simulink model "sampleModel182"  (R2021b)
settings: Solver=VariableStepAuto  StartTime=0.0  StopTime=10.0  RelTol=1e-3
undefined symbols (not defined in the file or in its folder): DiscIntNeverNeededParam
libraries: simulink x26, slpidlib x2, simulink_need_slupdate x2
settings Model: Creator=user  LastModifiedBy=user

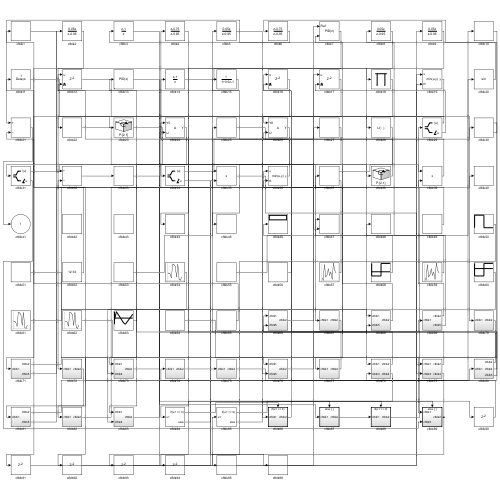
[thumbnail: Simulink's stored preview of the top-level diagram]
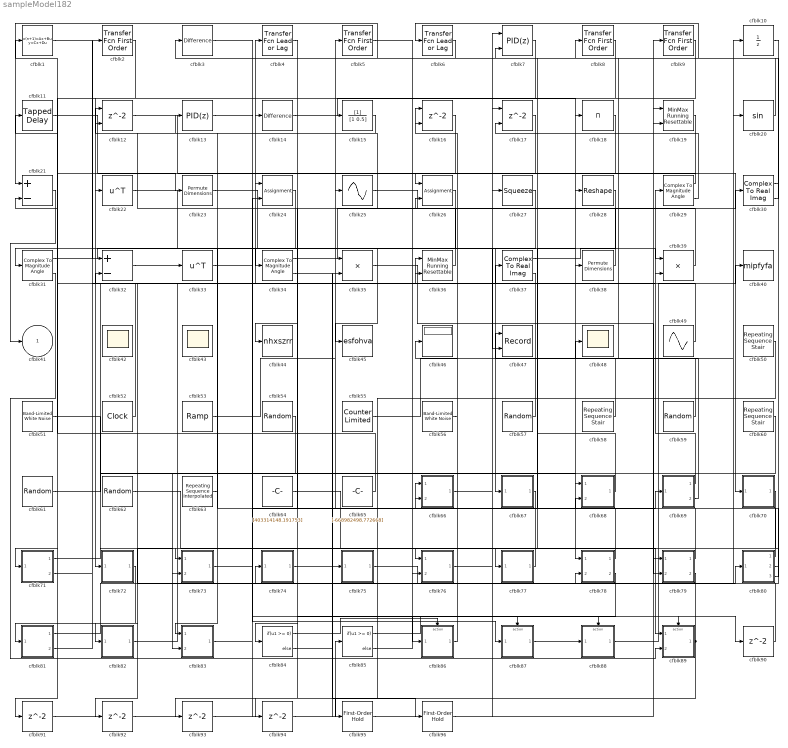
== system sampleModel182 ==
  cfblk1 : DiscreteStateSpace
  cfblk10 : UnitDelay  HasFrameUpgradeWarning=on
  cfblk11 : simulink/Discrete/Tapped Delay  vinit=0.0  samptime=-1  NumDelays=1  DelayOrder=Oldest  includeCurrent=off
  cfblk12 : Delay  ShowEnablePort=on  SampleTime=1
      settings: InputPortMap=u0,e6
  cfblk13 : slpidlib/PID Controller  Controller=PID  Form=Parallel  TimeDomain=Discrete-time  UseExternalTs=off  SampleTime=1  IntegratorMethod=Forward Euler  FilterMethod=Forward Euler  ControllerParametersSource=internal  P=1  I=1  D=0  UseFilter=on  N=100  TunerSelectOption=Transfer Function Based (PID Tuner App)  InitialConditionSource=internal  InitialConditionForIntegrator=0  InitialConditionForFilter=0  DifferentiatorICPrevScaledInput=0  ExternalReset=none  TrackingMode=off  Kt=1  LimitOutput=off  SatLimitsSource=internal  UpperSaturationLimit=inf  LowerSaturationLimit=-inf  LinearizeAsGain=off  AntiWindupMode=none  Kb=1  POutMin=[]  POutMax=[]  IOutMin=[]  IOutMax=[]  DOutMin=[]  DOutMax=[]  NOutMin=[]  NOutMax=[]  SumOutMin=[]  SumOutMax=[]  SaturationOutMin=[]  SaturationOutMax=[]  PParamMin=[]  PParamMax=[]  IParamMin=[]  IParamMax=[]  DParamMin=[]  DParamMax=[]  NParamMin=[]  NParamMax=[]  KbParamMin=[]  KbParamMax=[]  KtParamMin=[]  KtParamMax=[]  KbOutMin=[]  KbOutMax=[]  KtOutMin=[]  KtOutMax=[]  IntegratorOutMin=[]  IntegratorOutMax=[]  FilterOutMin=[]  FilterOutMax=[]  SumI1OutMin=[]  SumI1OutMax=[]  SumI2OutMin=[]  SumI2OutMax=[]  SumI3OutMin=[]  SumI3OutMax=[]  SumI4OutMin=[]  SumI4OutMax=[]  SumDOutMin=[]  SumDOutMax=[]  DifferentiatorOutMin=[]  DifferentiatorOutMax=[]  FilterDiffOutCoefMin=[]  FilterDiffOutCoefMax=[]  ReciprocalOutMin=[]  ReciprocalOutMax=[]  SumDenOutMin=[]  SumDenOutMax=[]  SumNumOutMin=[]  SumNumOutMax=[]  DivideOutMin=[]  DivideOutMax=[]  UdiffTsProdOutMin=[]  UdiffTsProdOutMax=[]  NTsProdOutMin=[]  NTsProdOutMax=[]  UintegralTsProdOutMin=[]  UintegralTsProdOutMax=[]  UngainTsProdOutMin=[]  UngainTsProdOutMax=[]  IntegratorContinuousStateAttributes=''  IntegratorStateMustResolveToSignalObject=off  IntegratorRTWStateStorageClass=Auto  FilterContinuousStateAttributes=''  FilterStateMustResolveToSignalObject=off  FilterRTWStateStorageClass=Auto  ParallelPVariant=InternalParameters  IdealPVariant=Disabled  IVariant=InternalParameters  DVariant=InternalParameters  IntegratorVariant=Discrete  SatVariant=Disabled  AWVariant=Passthrough  PCopyVariant=Disabled  TRVariant=Disabled  FdbkBlocksVariant=Forward  IdealPFdbkVariant=Disabled  SatFdbkVariant=Disabled  DerivativeFilterVariant=ForwardEulerFilter  NVariant=InternalParameters  NCopyVariant=Disabled  FilterICVariant=InternalICsFilter  IntegratorICVariant=InternalICs  ExternalResetVariant=Disabled  TRSumVariant=Passthrough  SumFdbkVariant=Disabled  SumVariant=Sum_PID  TsampFilterVariant=InternalTs  TsampNgainVariant=Passthrough  TsampIntegralVariant=Passthrough  ExternalSaturationOutDataTypeStr=Inherit: Same as second input
  cfblk14 : simulink/Discrete/Difference  ICPrevInput=0.0  OutMin=[]  OutMax=[]  OutDataTypeStr=Inherit: Inherit via back propagation  OutDataType=fixdt(1, 16)  OutScaling=2^-10  DoSatur=off
  cfblk15 : DiscreteFilter  SampleTime=1
  cfblk16 : Delay  ShowEnablePort=on  SampleTime=1
      settings: InputPortMap=u0,e6
  cfblk17 : Delay  ShowEnablePort=on  SampleTime=1
      settings: InputPortMap=u0,e6
  cfblk18 : Product  Inputs=*
  cfblk19 : simulink/Math Operations/MinMax Running Resettable  Function=min  vinit=0.0
  cfblk{2,5,8..9} (4 alike) : simulink/Discrete/Transfer Fcn First Order  PoleZ=0.95  ICPrevOutput=0.0  DoSatur=off
  cfblk20 : Trigonometry
  cfblk21 : Sum  Inputs=+-
  cfblk22 : Math  Operator=transpose  SaturateOnIntegerOverflow=on
  cfblk23 : PermuteDimensions
  cfblk24 : Assignment  DiagnosticForDimensions=Warning  IndexOptions=Index vector (dialog)  Indices=1  OutputSizes=1
  cfblk25 : Sin  TimeSource=Use external signal  SampleTime=0
  cfblk26 : Assignment  DiagnosticForDimensions=Warning  IndexOptions=Index vector (dialog)  Indices=1  OutputSizes=1
  cfblk27 : Squeeze
  cfblk28 : Reshape
  cfblk29 : ComplexToMagnitudeAngle
  cfblk3 : simulink/Discrete/Difference  ICPrevInput=0.0  OutMin=[]  OutMax=[]  OutDataTypeStr=Inherit: Inherit via back propagation  OutDataType=fixdt(1, 16)  OutScaling=2^-10  DoSatur=off
  cfblk30 : ComplexToRealImag
  cfblk31 : ComplexToMagnitudeAngle
  cfblk32 : Sum  Inputs=+-
  cfblk33 : Math  Operator=transpose  SaturateOnIntegerOverflow=on
  cfblk34 : ComplexToMagnitudeAngle
  cfblk35 : Product  Inputs=**
  cfblk36 : simulink/Math Operations/MinMax Running Resettable  Function=min  vinit=0.0
  cfblk37 : ComplexToRealImag
  cfblk38 : PermuteDimensions
  cfblk39 : Product
  cfblk4 : simulink/Discrete/Transfer Fcn Lead or Lag  PoleZ=0.95  ZeroZ=0.75  ICPrevOutput=0.0  ICPrevInput=0.0  DoSatur=off
      settings: SourceProductBaseCode=SL
  cfblk40 : ToWorkspace  VariableName=mipfyfa  SaveFormat=Timeseries  SampleTime=-1
  cfblk42 : Scope
      settings: Floating=on
  cfblk43 : Scope
      settings: Floating=on
  cfblk44 : ToWorkspace  VariableName=nhxszrr  SaveFormat=Timeseries  SampleTime=-1
  cfblk45 : ToWorkspace  VariableName=esfohva  SaveFormat=Timeseries  SampleTime=-1
  cfblk46 : Display
  cfblk47 : Record  FileSettingsInternal="{\"entries\":[{\"content\":{\"excelSettings\":{\"content\":{},\"type\":\"Streamout.ExcelSettings\"}},\"type\":\"Streamout.FileSettingStorage\",\"uuid\":\"d13ae737-717a-44e4-beef-aca473ab83c8\"}],\"packageUris\":[\"http://schema.mathworks.com/mf0/streamout_blocks/R2020a\"],\"version\":\"1.0\"}"  Layout=[1 1]  SignalsInternal="{\"entries\":[{\"content\":{\"signals\":[{\"content\":{\"blockPath\":[\"sampleModel182/cfblk47\"],\"channel\":[],\"dimensions\":[1],\"domain\":\"sampleModel182/cfblk47\",\"lineColor\":\"#a2142f\",\"plots\":[1],\"port\":1,\"sid\":[\"\"],\"signalID\":6832,\"signalName\":\"cfblk58\"},\"type\":\"RecordBlkView.Signal\",\"uuid\":\"52de0a0e-42b8-4ab6-a928-dbb1bce8dd43\"},{\"content\":{\"blockPath\":[\"sampleModel182/cfblk47\"],\"channel\":[],\"dimensions\":[1,1],\"domain\":\"sampleModel182/cfblk47\",\"lineColor\":\"#139fff\",\"plots\":[1],\"port\":2,\"sid\":[\"\"],\"signalID\":6836,\"signalName\":\"cfblk23\"},\"type\":\"RecordBlkView.Signal\",\"uuid\":\"73905647-726a-4450-a034-1e1480183f6b\"}]},\"type\":\"RecordBlkView.InputSignals\",\"uuid\":\"f9e11d63-c08c-4043-8374-cec281b00203\"}],\"packageUris\":[\"http://schema.mathworks.com/mf0/streamout_blocks/R2020a\"],\"version\":\"1.0\"}"  VisualizationBindings="{\"xyplotplugin\":{\"info\":[{\"series\":[{\"bindingParametersList\":[{\"parameter\":\"X-Axis\",\"signalID\":6832,\"signalName\":\"cfblk58\"},{\"parameter\":\"Y-Axis\",\"signalID\":6836,\"signalName\":\"cfblk23\"}],\"seriesID\":60133}],\"subplotID\":1}]}}"  CompatibilityTag=XY
  cfblk48 : Scope
  cfblk49 : Sin  Amplitude=[-141875672.299204]  Bias=[779859813.343924]  SampleTime=0
  cfblk50 : simulink/Sources/Repeating Sequence Stair  OutValues=[-60441637.723596, -585056576.833812]  tsamp=-1  OutMin=[]  OutMax=[]  OutDataTypeStr=double  OutputDataTypeScalingMode=double  OutDataType=fixdt(0,8)  ConRadixGroup=Best Precision: Vector-wise  OutScaling=2^-12
  cfblk51 : simulink/Sources/Band-Limited White Noise  Cov=[3530728018.912048]  Ts=0.1  seed=[8507991473.000000]
  cfblk52 : DigitalClock
  cfblk53 : simulink/Sources/Ramp  slope=[-7352.708295]  start=[35.890087]  InitialOutput=[746056.812358]
  cfblk54 : RandomNumber  Mean=[-75945.215518]  Variance=[96366.823792]  Seed=[128117105.000000]  SampleTime=0.1
  cfblk55 : simulink/Sources/Counter Limited  uplimit=[293.000000]  tsamp=-1
  cfblk56 : simulink/Sources/Band-Limited White Noise  Cov=[8244043055.109829]  Ts=0.1  seed=[8435438887.000000]
  cfblk57 : UniformRandomNumber  Minimum=[-2157205412.986696]  Maximum=[6030967556.197421]  Seed=[60259926.000000]  SampleTime=0.1
  cfblk58 : simulink/Sources/Repeating Sequence Stair  OutValues=[-406766921.722667, 853752626.696085]  tsamp=-1  OutMin=[]  OutMax=[]  OutDataTypeStr=double  OutputDataTypeScalingMode=double  OutDataType=fixdt(0,8)  ConRadixGroup=Best Precision: Vector-wise  OutScaling=2^-12
  cfblk59 : UniformRandomNumber  Minimum=[-1472469171.616397]  Maximum=[7630143098.593646]  Seed=[576780.000000]  SampleTime=0.1
  cfblk6 : simulink/Discrete/Transfer Fcn Lead or Lag  PoleZ=0.95  ZeroZ=0.75  ICPrevOutput=0.0  ICPrevInput=0.0  DoSatur=off
      settings: SourceProductBaseCode=SL
  cfblk60 : simulink/Sources/Repeating Sequence Stair  OutValues=[-994952748.638581, 736349140.232044]  tsamp=-1  OutMin=[]  OutMax=[]  OutDataTypeStr=double  OutputDataTypeScalingMode=double  OutDataType=fixdt(0,8)  ConRadixGroup=Best Precision: Vector-wise  OutScaling=2^-12
  cfblk61 : RandomNumber  Mean=[-83719.309304]  Variance=[73957.021569]  Seed=[698296596.000000]  SampleTime=0.1
  cfblk62 : RandomNumber  Mean=[-58692.559989]  Variance=[72148.805861]  Seed=[413759557.000000]  SampleTime=0.1
  cfblk63 : simulink/Sources/Repeating Sequence Interpolated  OutValues=[-173788248.705158, 694979924.956819, -526378748.977150, -611525270.001202, 418441487.960879]  TimeValues=[0 0.1 0.5 0.6 1].'  LookUpMeth=Use Input Above  tsamp=0.01  OutMin=[]  OutMax=[]  OutDataTypeStr=double  OutputDataTypeScalingMode=double  OutDataType=fixdt(0,8)  OutScaling=2^-10
  cfblk64 : Constant  Value=[403314148.191753]  SampleTime=1
  cfblk65 : Constant  Value=[-668982498.772668]  SampleTime=1
  cfblk66 : Subsystem
  cfblk67 : Subsystem
  cfblk68 : Subsystem
  cfblk69 : Subsystem
  cfblk7 : slpidlib/PID Controller (2DOF)  Controller=PID  Form=Parallel  TimeDomain=Discrete-time  UseExternalTs=off  SampleTime=1  IntegratorMethod=Forward Euler  FilterMethod=Forward Euler  ControllerParametersSource=internal  P=1  I=1  D=0  UseFilter=on  N=100  b=1  c=1  TunerSelectOption=Transfer Function Based (PID Tuner App)  InitialConditionSource=internal  InitialConditionForIntegrator=0  InitialConditionForFilter=0  DifferentiatorICPrevScaledInput=0  ExternalReset=none  TrackingMode=off  Kt=1  LimitOutput=off  SatLimitsSource=internal  UpperSaturationLimit=inf  LowerSaturationLimit=-inf  LinearizeAsGain=off  AntiWindupMode=none  Kb=1  POutMin=[]  POutMax=[]  IOutMin=[]  IOutMax=[]  DOutMin=[]  DOutMax=[]  NOutMin=[]  NOutMax=[]  bOutMin=[]  bOutMax=[]  cOutMin=[]  cOutMax=[]  SumOutMin=[]  SumOutMax=[]  SaturationOutMin=[]  SaturationOutMax=[]  PParamMin=[]  PParamMax=[]  IParamMin=[]  IParamMax=[]  DParamMin=[]  DParamMax=[]  NParamMin=[]  NParamMax=[]  bParamMin=[]  bParamMax=[]  cParamMin=[]  cParamMax=[]  KbParamMin=[]  KbParamMax=[]  KtParamMin=[]  KtParamMax=[]  KbOutMin=[]  KbOutMax=[]  KtOutMin=[]  KtOutMax=[]  IntegratorOutMin=[]  IntegratorOutMax=[]  FilterOutMin=[]  FilterOutMax=[]  SumI1OutMin=[]  SumI1OutMax=[]  SumI2OutMin=[]  SumI2OutMax=[]  SumI3OutMin=[]  SumI3OutMax=[]  SumI4OutMin=[]  SumI4OutMax=[]  SumDOutMin=[]  SumDOutMax=[]  Sum1OutMin=[]  Sum1OutMax=[]  Sum2OutMin=[]  Sum2OutMax=[]  Sum3OutMin=[]  Sum3OutMax=[]  DifferentiatorOutMin=[]  DifferentiatorOutMax=[]  FilterDiffOutCoefMin=[]  FilterDiffOutCoefMax=[]  ReciprocalOutMin=[]  ReciprocalOutMax=[]  SumDenOutMin=[]  SumDenOutMax=[]  SumNumOutMin=[]  SumNumOutMax=[]  DivideOutMin=[]  DivideOutMax=[]  UdiffTsProdOutMin=[]  UdiffTsProdOutMax=[]  NTsProdOutMin=[]  NTsProdOutMax=[]  UintegralTsProdOutMin=[]  UintegralTsProdOutMax=[]  UngainTsProdOutMin=[]  UngainTsProdOutMax=[]  IntegratorContinuousStateAttributes=''  IntegratorStateMustResolveToSignalObject=off  IntegratorRTWStateStorageClass=Auto  FilterContinuousStateAttributes=''  FilterStateMustResolveToSignalObject=off  FilterRTWStateStorageClass=Auto  ParallelPVariant=InternalParameters  IdealPVariant=Disabled  IVariant=InternalParameters  DVariant=InternalParameters  bVariant=InternalParameters  cVariant=InternalParameters  IntegratorVariant=Discrete  SatVariant=Disabled  AWVariant=Passthrough  PCopyVariant=Disabled  TRVariant=Disabled  FdbkBlocksVariant=Forward  IdealPFdbkVariant=Disabled  SatFdbkVariant=Disabled  DerivativeFilterVariant=ForwardEulerFilter  NVariant=InternalParameters  NCopyVariant=Disabled  FilterICVariant=InternalICsFilter  IntegratorICVariant=InternalICs  ExternalResetVariant=Disabled  TRSumVariant=Passthrough  SumFdbkVariant=Disabled  SumVariant=Sum_PID  TsampFilterVariant=InternalTs  TsampNgainVariant=Passthrough  TsampIntegralVariant=Passthrough  ExternalSaturationOutDataTypeStr=Inherit: Same as second input
      settings: SourceProductBaseCode=SL
  cfblk70 : Subsystem
  cfblk71 : Subsystem
  cfblk72 : Subsystem
  cfblk73 : Subsystem
  cfblk74 : Subsystem
  cfblk75 : Subsystem
  cfblk76 : Subsystem
  cfblk77 : Subsystem
  cfblk78 : Subsystem
  cfblk79 : Subsystem
  cfblk80 : Subsystem
  cfblk81 : Subsystem
  cfblk82 : Subsystem
  cfblk83 : Subsystem
  cfblk84 : If  IfExpression=u1 >= 0  SampleTime=1
  cfblk85 : If  IfExpression=u1 >= 0  SampleTime=1
  cfblk86 : Subsystem  TreatAsAtomicUnit=on
  cfblk87 : Subsystem  TreatAsAtomicUnit=on
  cfblk88 : Subsystem  TreatAsAtomicUnit=on
  cfblk89 : Subsystem  TreatAsAtomicUnit=on
  cfblk{90..94} (5 alike) : Delay  SampleTime=1
  cfblk95 : simulink_need_slupdate/First-Order Hold  DisableCoverage=on  Ts=1
      settings: SourceProductBaseCode=SL
  cfblk96 : simulink_need_slupdate/First-Order Hold  DisableCoverage=on  Ts=1
      settings: SourceProductBaseCode=SL
  cfblk41 : Outport
  wires:
  cfblk24/1 -> cfblk31/1
  cfblk2/1 -> cfblk72/1(cfblk1)
  cfblk12/1 -> cfblk70/1(cfblk1)
  cfblk62/1 -> cfblk76/1(cfblk1)
  cfblk32/1 -> cfblk33/1
  cfblk10/1 -> cfblk74/1(cfblk1)
  cfblk19/1 -> cfblk26/1
  cfblk22/1 -> cfblk67/1(cfblk1)
  cfblk28/1 -> cfblk77/1(cfblk1)
  cfblk67/1(cfblk2) -> cfblk81/1(cfblk1)
  cfblk9/1 -> cfblk78/1(cfblk1)
  cfblk21/1 -> cfblk41/1
  cfblk82/1(cfblk2) -> cfblk4/1
  cfblk75/1(cfblk2) -> cfblk80/1(cfblk1)
  cfblk20/1 -> cfblk6/1
  cfblk29/1 -> cfblk22/1
  cfblk88/1(cfblk2) -> cfblk40/1
  cfblk49/1 -> cfblk16/1
  cfblk89/1(cfblk2) -> cfblk16/2, cfblk93/1
  cfblk74/1(cfblk2) -> cfblk75/1(cfblk1)
  cfblk27/1 -> cfblk73/1(cfblk1)
  cfblk87/1(cfblk2) -> cfblk88/1(cfblk1)
  cfblk63/1 -> cfblk13/1
  cfblk18/1 -> cfblk28/1
  cfblk66/1(cfblk2) -> cfblk27/1
  cfblk78/1(cfblk2) -> cfblk5/1
  cfblk53/1 -> cfblk25/1
  cfblk54/1 -> cfblk83/1(cfblk1)
  cfblk38/1 -> cfblk14/1
  cfblk51/1 -> cfblk68/1(cfblk1)
  cfblk69/1(cfblk2) -> cfblk29/1
  cfblk25/1 -> cfblk30/1
  cfblk16/1 -> cfblk76/2(cfblk5)
  cfblk64/1 -> cfblk89/1(cfblk1)
  cfblk4/1 -> cfblk44/1
  cfblk55/1 -> cfblk10/1
  cfblk8/1 -> cfblk84/1
  cfblk6/1 -> cfblk21/1
  cfblk11/1 -> cfblk23/1
  cfblk86/1(cfblk2) -> cfblk46/1
  cfblk69/2(cfblk5) -> cfblk48/1
  cfblk52/1 -> cfblk1/1
  cfblk80/1(cfblk2) -> cfblk37/1
  cfblk3/1 -> cfblk87/1(cfblk1)
  cfblk76/1(cfblk2) -> cfblk69/1(cfblk1)
  cfblk59/1 -> cfblk8/1
  cfblk61/1 -> cfblk9/1
  cfblk77/1(cfblk2) -> cfblk36/1
  cfblk34/1 -> cfblk17/1
  cfblk80/2(cfblk4) -> cfblk66/1(cfblk1)
  cfblk79/1(cfblk2) -> cfblk24/1
  cfblk39/1 -> cfblk12/1
  cfblk5/1 -> cfblk86/1(cfblk1)
  cfblk56/1 -> cfblk26/2
  cfblk15/1 -> cfblk12/2
  cfblk60/1 -> cfblk83/2(cfblk4)
  cfblk65/1 -> cfblk11/1
  cfblk73/1(cfblk2) -> cfblk35/1
  cfblk14/1 -> cfblk18/1
  cfblk81/1(cfblk2) -> cfblk20/1
  cfblk36/1 -> cfblk15/1
  cfblk37/1 -> cfblk39/1
  cfblk83/1(cfblk2) -> cfblk68/2(cfblk5)
  cfblk79/2(cfblk4) -> cfblk78/2(cfblk3)
  cfblk58/1 -> cfblk47/1
  cfblk71/1(cfblk2) -> cfblk73/2(cfblk4)
  cfblk57/1 -> cfblk21/2
  cfblk35/1 -> cfblk79/1(cfblk1)
  cfblk26/1 -> cfblk45/1
  cfblk31/1 -> cfblk34/1
  cfblk29/2 -> cfblk17/2
  cfblk80/3(cfblk5) -> cfblk66/2(cfblk5)
  cfblk31/2 -> cfblk89/2(cfblk5)
  cfblk72/1(cfblk2) -> cfblk82/1(cfblk1)
  cfblk37/2 -> cfblk36/2
  cfblk71/2(cfblk5) -> cfblk2/1
  cfblk68/1(cfblk2) -> cfblk7/2
  cfblk30/1 -> cfblk79/2(cfblk3)
  cfblk30/2 -> cfblk3/1
  cfblk7/1 -> cfblk71/1(cfblk1)
  cfblk1/1 -> cfblk32/1
  cfblk13/1 -> cfblk38/1
  cfblk81/2(cfblk5) -> cfblk39/2
  cfblk23/1 -> cfblk47/2
  cfblk84/1 -> cfblk86/Action
  cfblk84/2 -> cfblk87/Action
  cfblk85/1 -> cfblk88/Action
  cfblk85/2 -> cfblk89/Action
  cfblk33/1 -> cfblk90/1
  cfblk90/1 -> cfblk32/2
  cfblk17/1 -> cfblk91/1
  cfblk91/1 -> cfblk35/2
  cfblk70/1(cfblk2) -> cfblk92/1
  cfblk92/1 -> cfblk85/1
  cfblk93/1 -> cfblk24/2
  cfblk78/2(cfblk4) -> cfblk94/1
  cfblk94/1 -> cfblk7/1
  cfblk50/1 -> cfblk95/1
  cfblk95/1 -> cfblk19/1
  cfblk34/2 -> cfblk96/1
  cfblk96/1 -> cfblk19/2

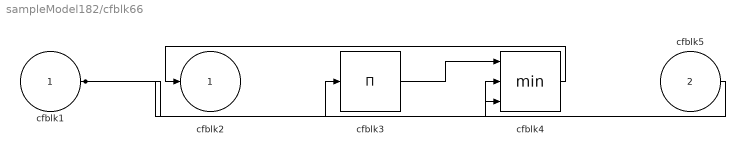
== system sampleModel182/cfblk66 ==
  cfblk1 : Inport
  cfblk5 : Inport  Port=2
  cfblk3 : Product  Inputs=*
  cfblk4 : MinMax  Inputs=3
  cfblk2 : Outport
  wires:
  cfblk4/1 -> cfblk2/1
  cfblk1/1 -> cfblk3/1, cfblk4/3
  cfblk3/1 -> cfblk4/1
  cfblk5/1 -> cfblk4/2

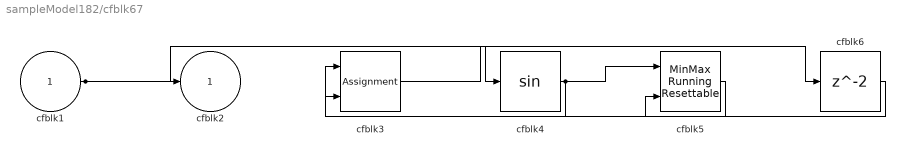
== system sampleModel182/cfblk67 ==
  cfblk1 : Inport
  cfblk3 : Assignment  DiagnosticForDimensions=Warning  IndexOptions=Index vector (dialog)  Indices=1  OutputSizes=1
  cfblk4 : Trigonometry
  cfblk5 : simulink/Math Operations/MinMax Running Resettable  Function=min  vinit=0.0
  cfblk6 : Delay  SampleTime=1
  cfblk2 : Outport
  wires:
  cfblk1/1 -> cfblk4/1, cfblk2/1
  cfblk5/1 -> cfblk3/1
  cfblk4/1 -> cfblk5/1, cfblk3/2
  cfblk3/1 -> cfblk6/1
  cfblk6/1 -> cfblk5/2

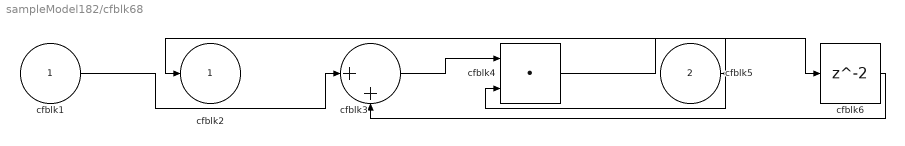
== system sampleModel182/cfblk68 ==
  cfblk1 : Inport
  cfblk5 : Inport  Port=2
  cfblk3 : Sum  Inputs=|++
  cfblk4 : DotProduct  InputSameDT=on  OutDataTypeStr=Inherit: Inherit via internal rule
  cfblk6 : Delay  SampleTime=1
  cfblk2 : Outport
  wires:
  cfblk5/1 -> cfblk2/1, cfblk4/2
  cfblk1/1 -> cfblk3/1
  cfblk3/1 -> cfblk4/1
  cfblk4/1 -> cfblk6/1
  cfblk6/1 -> cfblk3/2

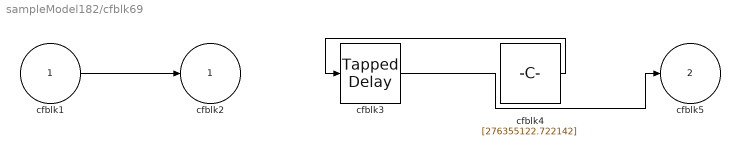
== system sampleModel182/cfblk69 ==
  cfblk1 : Inport
  cfblk3 : simulink/Discrete/Tapped Delay  vinit=0.0  samptime=-1  NumDelays=1  DelayOrder=Oldest  includeCurrent=off
  cfblk4 : Constant  Value=[276355122.722142]  SampleTime=1
  cfblk2 : Outport
  cfblk5 : Outport  Port=2
  wires:
  cfblk4/1 -> cfblk3/1
  cfblk3/1 -> cfblk5/1
  cfblk1/1 -> cfblk2/1

== system sampleModel182/cfblk70 ==
  cfblk1 : Inport
  cfblk3 : Sum  Inputs=+-
  cfblk4 : Assignment  DiagnosticForDimensions=Warning  IndexOptions=Index vector (dialog)  Indices=1  OutputSizes=1
  cfblk2 : Outport
  wires:
  cfblk3/1 -> cfblk2/1
  cfblk1/1 -> cfblk3/1, cfblk4/1, cfblk4/2
  cfblk4/1 -> cfblk3/2

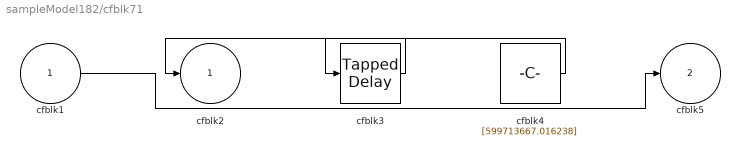
== system sampleModel182/cfblk71 ==
  cfblk1 : Inport
  cfblk3 : simulink/Discrete/Tapped Delay  vinit=0.0  samptime=-1  NumDelays=1  DelayOrder=Oldest  includeCurrent=off
  cfblk4 : Constant  Value=[599713667.016238]  SampleTime=1
  cfblk2 : Outport
  cfblk5 : Outport  Port=2
  wires:
  cfblk3/1 -> cfblk2/1
  cfblk1/1 -> cfblk5/1
  cfblk4/1 -> cfblk3/1

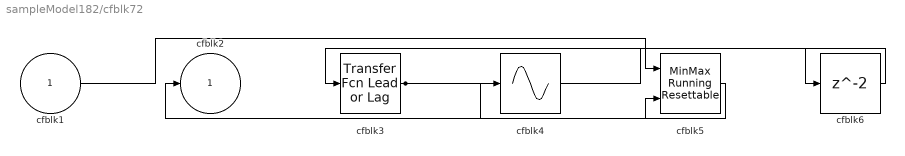
== system sampleModel182/cfblk72 ==
  cfblk1 : Inport
  cfblk3 : simulink/Discrete/Transfer Fcn Lead or Lag  PoleZ=0.95  ZeroZ=0.75  ICPrevOutput=0.0  ICPrevInput=0.0  DoSatur=off
      settings: SourceProductBaseCode=SL
  cfblk4 : Sin  TimeSource=Use external signal  SampleTime=0
  cfblk5 : simulink/Math Operations/MinMax Running Resettable  Function=min  vinit=0.0
  cfblk6 : Delay  SampleTime=1
  cfblk2 : Outport
  wires:
  cfblk3/1 -> cfblk4/1, cfblk5/2
  cfblk5/1 -> cfblk2/1
  cfblk1/1 -> cfblk5/1
  cfblk4/1 -> cfblk6/1
  cfblk6/1 -> cfblk3/1

== system sampleModel182/cfblk73 ==
  cfblk1 : Inport
  cfblk4 : Inport  Port=2
  cfblk3 : Constant  Value=[76629421.829974]  SampleTime=1
  cfblk2 : Outport
  wires:
  cfblk4/1 -> cfblk2/1

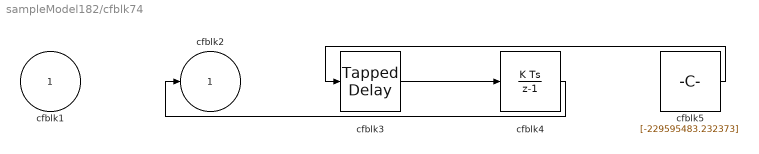
== system sampleModel182/cfblk74 ==
  cfblk1 : Inport
  cfblk3 : simulink/Discrete/Tapped Delay  vinit=0.0  samptime=-1  NumDelays=1  DelayOrder=Oldest  includeCurrent=off
  cfblk4 : DiscreteIntegrator  ICPrevOutput=DiscIntNeverNeededParam  ICPrevScaledInput=DiscIntNeverNeededParam
  cfblk5 : Constant  Value=[-229595483.232373]  SampleTime=1
  cfblk2 : Outport
  wires:
  cfblk5/1 -> cfblk3/1
  cfblk4/1 -> cfblk2/1
  cfblk3/1 -> cfblk4/1

== system sampleModel182/cfblk75 ==
  cfblk1 : Inport
  cfblk3 : Bias  Bias=[-987009397.239793]
  cfblk2 : Outport
  wires:
  cfblk3/1 -> cfblk2/1
  cfblk1/1 -> cfblk3/1

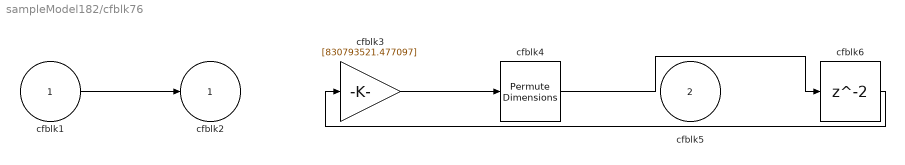
== system sampleModel182/cfblk76 ==
  cfblk1 : Inport
  cfblk5 : Inport  Port=2
  cfblk3 : Gain  Gain=[830793521.477097]
  cfblk4 : PermuteDimensions
  cfblk6 : Delay  SampleTime=1
  cfblk2 : Outport
  wires:
  cfblk3/1 -> cfblk4/1
  cfblk1/1 -> cfblk2/1
  cfblk4/1 -> cfblk6/1
  cfblk6/1 -> cfblk3/1

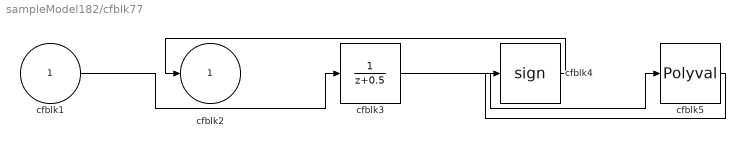
== system sampleModel182/cfblk77 ==
  cfblk1 : Inport
  cfblk3 : DiscreteTransferFcn  SampleTime=1
  cfblk4 : Signum
  cfblk5 : Polyval  Coefs=[ +2.081618890e-019, -1.441693666e-014, +4.719686976e-010, -8.536869453e-006, +1.621573104e-001, -8.087801117e+001 ]
  cfblk2 : Outport
  wires:
  cfblk4/1 -> cfblk2/1
  cfblk1/1 -> cfblk3/1
  cfblk3/1 -> cfblk5/1
  cfblk5/1 -> cfblk4/1

== system sampleModel182/cfblk78 ==
  cfblk1 : Inport
  cfblk3 : Inport  Port=2
  cfblk2 : Outport
  cfblk4 : Outport  Port=2
  wires:
  cfblk3/1 -> cfblk2/1
  cfblk1/1 -> cfblk4/1

== system sampleModel182/cfblk79 ==
  cfblk1 : Inport
  cfblk3 : Inport  Port=2
  cfblk2 : Outport
  cfblk4 : Outport  Port=2
  wires:
  cfblk1/1 -> cfblk2/1
  cfblk3/1 -> cfblk4/1

== system sampleModel182/cfblk80 ==
  cfblk1 : Inport
  cfblk3 : Constant  Value=[480534822.237800]  SampleTime=1
  cfblk2 : Outport
  cfblk4 : Outport  Port=2
  cfblk5 : Outport  Port=3
  wires:
  cfblk3/1 -> cfblk5/1
  cfblk1/1 -> cfblk2/1, cfblk4/1

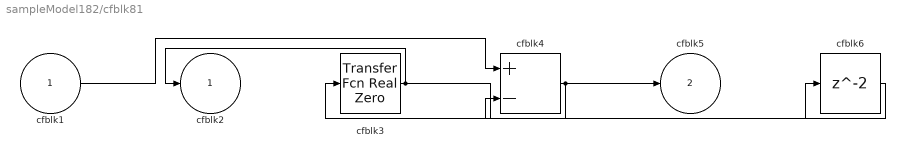
== system sampleModel182/cfblk81 ==
  cfblk1 : Inport
  cfblk3 : simulink/Discrete/Transfer Fcn Real Zero  ZeroZ=0.75  ICPrevInput=0.0  DoSatur=off
      settings: SourceProductBaseCode=SL
  cfblk4 : Sum  Inputs=+-
  cfblk6 : Delay  SampleTime=1
  cfblk2 : Outport
  cfblk5 : Outport  Port=2
  wires:
  cfblk3/1 -> cfblk2/1, cfblk6/1
  cfblk1/1 -> cfblk4/1
  cfblk4/1 -> cfblk3/1, cfblk5/1
  cfblk6/1 -> cfblk4/2

== system sampleModel182/cfblk82 ==
  cfblk1 : Inport
  cfblk3 : ComplexToRealImag
  cfblk2 : Outport
  wires:
  cfblk3/1 -> cfblk2/1
  cfblk1/1 -> cfblk3/1

== system sampleModel182/cfblk83 ==
  cfblk1 : Inport
  cfblk4 : Inport  Port=2
  cfblk3 : MinMax  Function=max  Inputs=2
  cfblk2 : Outport
  wires:
  cfblk4/1 -> cfblk3/1
  cfblk1/1 -> cfblk3/2
  cfblk3/1 -> cfblk2/1

== system sampleModel182/cfblk86 ==
  cfblk1 : Inport
  Action Port : ActionPort  ActionPortLabel=if(u1 >= 0)
  cfblk3 : Abs
  cfblk4 : Reshape
  cfblk2 : Outport
  wires:
  cfblk3/1 -> cfblk2/1
  cfblk4/1 -> cfblk3/1
  cfblk1/1 -> cfblk4/1

== system sampleModel182/cfblk87 ==
  cfblk1 : Inport
  Action Port : ActionPort  ActionPortLabel=else
  cfblk3 : Reshape
  cfblk2 : Outport
  wires:
  cfblk1/1 -> cfblk3/1
  cfblk3/1 -> cfblk2/1

== system sampleModel182/cfblk88 ==
  cfblk1 : Inport
  Action Port : ActionPort  ActionPortLabel=if(u1 >= 0)
  cfblk3 : Signum
  cfblk2 : Outport
  wires:
  cfblk1/1 -> cfblk3/1
  cfblk3/1 -> cfblk2/1

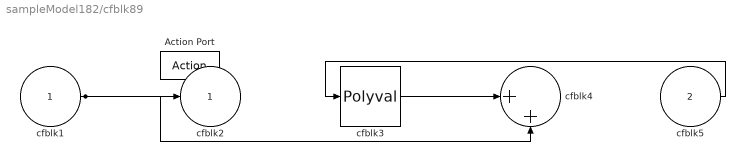
== system sampleModel182/cfblk89 ==
  cfblk1 : Inport
  cfblk5 : Inport  Port=2
  Action Port : ActionPort  ActionPortLabel=else
  cfblk3 : Polyval  Coefs=[ +2.081618890e-019, -1.441693666e-014, +4.719686976e-010, -8.536869453e-006, +1.621573104e-001, -8.087801117e+001 ]
  cfblk4 : Sum  Inputs=|++
  cfblk2 : Outport
  wires:
  cfblk5/1 -> cfblk3/1
  cfblk1/1 -> cfblk2/1, cfblk4/2
  cfblk3/1 -> cfblk4/1
